simulink model "Kapila"  (R2022b)
settings: Solver=VariableStepAuto  StartTime=0.0  StopTime=15  RelTol=1e-3
settings Model: Creator=Jared Stewart  LastModifiedBy=Jared Stewart

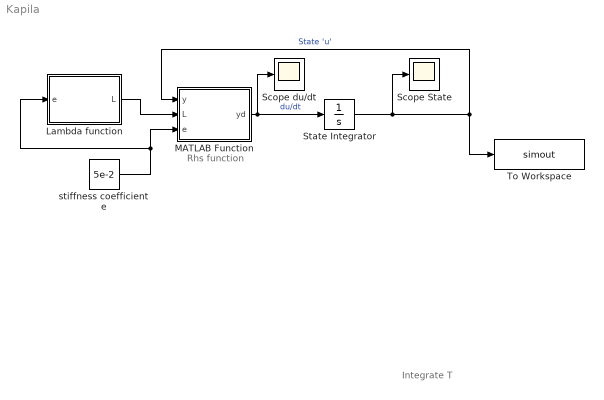
== system Kapila ==
  note: Rhs function
  note: Integrate T
  Lambda function : MATLAB Function  TreatAsAtomicUnit=on
  MATLAB Function : MATLAB Function  TreatAsAtomicUnit=on
  Scope State : Scope
  Scope du/dt : Scope
  State Integrator : Integrator  InitialCondition=[1;0.995;0.005]  AbsoluteTolerance=1e-4
  To Workspace : ToWorkspace  VariableName=simout  SaveFormat=Timeseries  SampleTime=-1
  stiffness coefficient  e : Constant  Value=5e-2
  wires:
  MATLAB Function/1(yd) -> State Integrator/1, Scope du/dt/1  "du/dt"
  State Integrator/1 -> MATLAB Function/1(y), To Workspace/1, Scope State/1  "State 'u'"
  stiffness coefficient  e/1 -> Lambda function/1(e), MATLAB Function/3(e)
  Lambda function/1(L) -> MATLAB Function/2(L)

== matlab function Kapila/Lambda function ==
  data: e input; L output
function L = L(e)
%ToDo:  Compute the lambda value for the simulation.  Remember the
%stiffness coefficient varies.
L = exp(1/e);

== matlab function Kapila/MATLAB Function ==
  data: y input; yd output; L input; e input
function yd=rhs(y,L,e)
    %ToDo: Write a system of ODEs (see Kapila's "Homogeneous branched-chain
    %explosion: Initiation to completion")
    yd=zeros(3,1);
    %L
    omega=L*y(2).*y(3).*exp(-1./(e*y(1)));
    %omega
    yd(1)=y(3);
    yd(2)=-omega;
    yd(3)=-yd(2)-yd(1);
